simulink model "st2"  (R2018b)
settings: Solver=VariableStepAuto  StartTime=0.0  StopTime=10.0  RelTol=1e-3
settings Model: Creator=12732  LastModifiedBy=12732

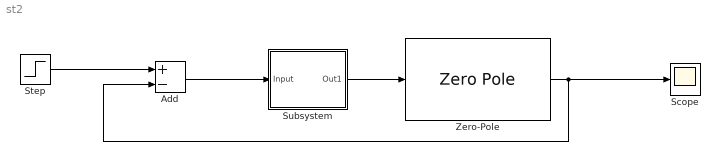
== system st2 ==
  Add : Sum  Inputs=+-
  Scope : Scope
  Step : Step  SampleTime=0
  Subsystem : Subsystem  mask{Kp=11.520, Ti=0.658, N=1, Td=0.164}
  Zero-Pole : ZeroPole  Zeros=[]  Poles=[-1 -3 -5]  Gain=2
  wires:
  Zero-Pole/1 -> Add/2, Scope/1
  Step/1 -> Add/1
  Add/1 -> Subsystem/1(Input)
  Subsystem/1(Out1) -> Zero-Pole/1

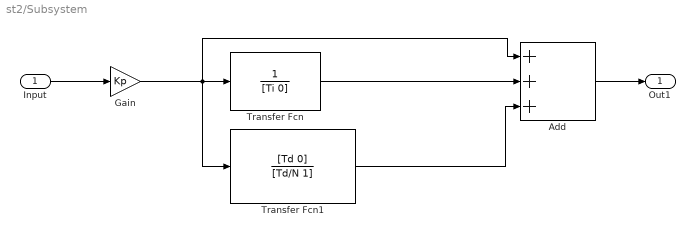
== system st2/Subsystem ==
  Input : Inport
  Add : Sum  Inputs=+++
  Gain : Gain  Gain=Kp
  Transfer Fcn : TransferFcn  Denominator=[Ti 0]
  Transfer Fcn1 : TransferFcn  Numerator=[Td 0]  Denominator=[Td/N 1]
  Out1 : Outport
  wires:
  Add/1 -> Out1/1
  Input/1 -> Gain/1
  Gain/1 -> Transfer Fcn1/1, Transfer Fcn/1, Add/1
  Transfer Fcn/1 -> Add/2
  Transfer Fcn1/1 -> Add/3
